simulink model "P3S"  (R2025b)
settings: Solver=VariableStepAuto  StartTime=0.0  StopTime=10.0  RelTol=1e-3
values from neighbouring files (symbols this model uses):
  b1 = 1000    [P3C.m]    (also in PR3.m)
  dx1 = 0    [P3C.m]
  dx2 = 0    [P3C.m]
  f = 0    [P3C.m]    (also in PR3.m)
  k1 = 16182    [P3C.m]    (also in PR3.m)
  k2 = 19000    [P3C.m]    (also in PR3.m)
  m1 = 290    [P3C.m]    (also in PR3.m)
  m2 = 59    [P3C.m]    (also in PR3.m)
  x1 = 0    [P3C.m]
  x2 = 0    [P3C.m]
settings Model: Creator=juani  LastModifiedBy=juani

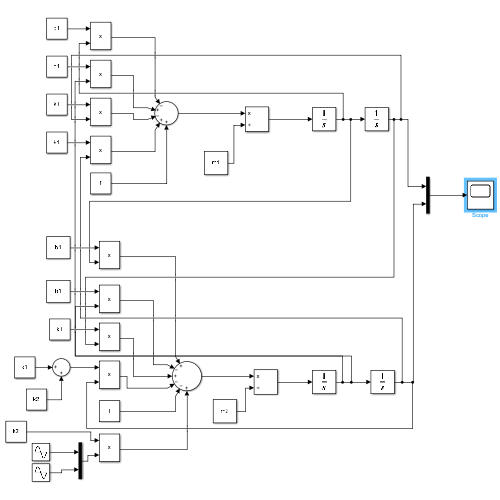
[thumbnail: Simulink's stored preview of the top-level diagram]
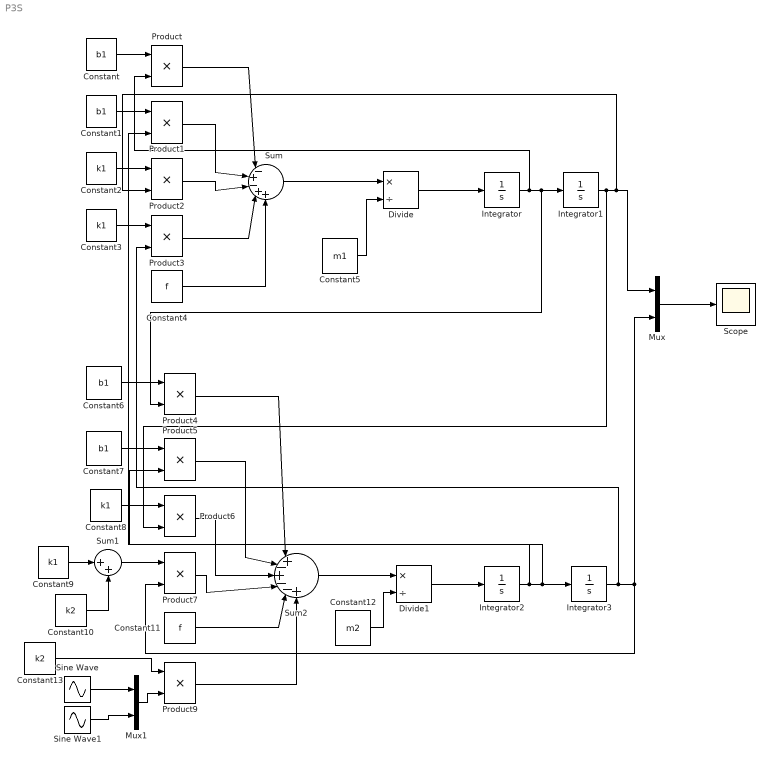
== system P3S ==
  Constant{,1,6..7} (4 alike) : Constant  Value=b1
  Constant10 : Constant  Value=k2
  Constant11 : Constant  Value=f
  Constant12 : Constant  Value=m2
  Constant13 : Constant  Value=k2
  Constant{2..3,8..9} (4 alike) : Constant  Value=k1
  Constant4 : Constant  Value=f
  Constant5 : Constant  Value=m1
  Divide : Product  Inputs=*/
  Divide1 : Product  Inputs=*/
  Integrator : Integrator  InitialCondition=dx1
  Integrator1 : Integrator  InitialCondition=x1
  Integrator2 : Integrator  InitialCondition=dx2
  Integrator3 : Integrator  InitialCondition=x2
  Mux : Mux  Inputs=2
  Mux1 : Mux  Inputs=2
  Product{,1..7,9} (9 alike) : Product
  Scope : Scope
      settings: ActiveDisplayYMinimum=-0.0702441559438079  ActiveDisplayYMaximum=0.080568186773229647
  Sine Wave : Sin  Amplitude=0.05  Frequency=0.5*pi  SampleTime=0
  Sine Wave1 : Sin  Amplitude=0.05  Frequency=20*pi  SampleTime=0
  Sum : Sum  Inputs=|-+-++
  Sum1 : Sum  Inputs=|++
  Sum2 : Sum  Inputs=|+-+--+
  wires:
  Constant/1 -> Product/1
  Constant1/1 -> Product1/1
  Constant2/1 -> Product2/1
  Constant3/1 -> Product3/1
  Product/1 -> Sum/1
  Product1/1 -> Sum/2
  Product2/1 -> Sum/3
  Product3/1 -> Sum/4
  Constant4/1 -> Sum/5
  Constant5/1 -> Divide/2
  Sum/1 -> Divide/1
  Integrator/1 -> Product/2, Product4/2, Integrator1/1
  Divide/1 -> Integrator/1
  Integrator1/1 -> Product6/2, Product2/2, Mux/1
  Constant6/1 -> Product4/1
  Constant7/1 -> Product5/1
  Constant8/1 -> Product6/1
  Constant9/1 -> Sum1/1
  Constant10/1 -> Sum1/2
  Sum1/1 -> Product7/1
  Mux1/1 -> Product9/2
  Sine Wave/1 -> Mux1/1
  Sine Wave1/1 -> Mux1/2
  Constant13/1 -> Product9/1
  Product4/1 -> Sum2/1
  Product5/1 -> Sum2/2
  Product6/1 -> Sum2/3
  Product7/1 -> Sum2/4
  Constant11/1 -> Sum2/5
  Product9/1 -> Sum2/6
  Sum2/1 -> Divide1/1
  Constant12/1 -> Divide1/2
  Divide1/1 -> Integrator2/1
  Integrator2/1 -> Product1/2, Product5/2, Integrator3/1
  Integrator3/1 -> Product3/2, Product7/2, Mux/2
  Mux/1 -> Scope/1
